simulink model "a1e1"  (R2020a)
settings: Solver=VariableStepAuto  StartTime=0.0  StopTime=200  RelTol=1e-3
settings Model: Creator=vivek vivian  LastModifiedBy=vivek vivian

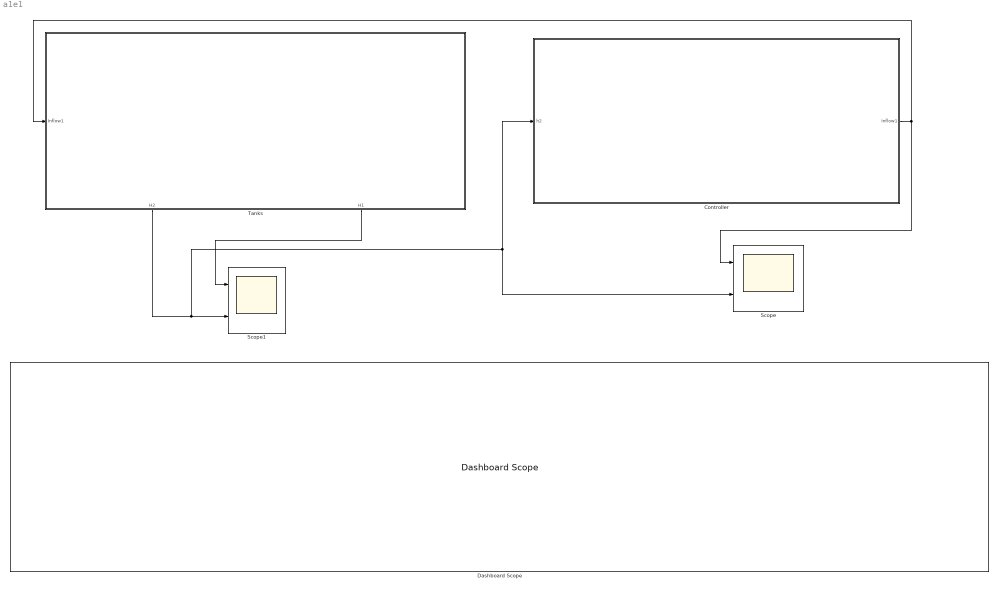
== system a1e1 ==
  Controller : Subsystem
  Dashboard Scope : DashboardScope
  Scope : Scope  NumInputPorts=2
  Scope1 : Scope  NumInputPorts=2
  Tanks : Subsystem
      settings: PortSchema="{\"entries\":[{\"content\":{\"sides\":[{\"content\":{\"connectorIds\":[\"In1\"]},\"type\":\"ConnectorPlacement.EquallySpacedRectSide\",\"uuid\":\"e5306d54-3110-4a08-a7f7-5a5ae3387896\"},{\"content\":{\"connectorIds\":[],\"side\":\"RIGHT\"},\"type\":\"ConnectorPlacement.EquallySpacedRectSide\",\"uuid\":\"42eaa8c0-5f21-4179-a706-71b62f07686c\"},{\"content\":{\"connectorIds\":[],\"side\":\"TOP\"},\"type\":\"ConnectorPlacement.EquallySpacedRectSide\",\"uuid\":\"3c777650-c00c-4d8d-89ca-bf2a69e675bf\"},{\"content\":{\"connectorIds\":[\"Out1\",\"Out2\"],\"side\":\"BOTTOM\"},\"type\":\"ConnectorPlacement.EquallySpacedRectSide\",\"uuid\":\"c8daac80-6471-486d-b612-ea006b4d9ffc\"}]},\"type\":\"ConnectorPlacement.EquallySpacedConnector\",\"uuid\":\"5a7e1e9a-909c-4566-afd0-a9330854ec0a\"}],\"packageUris\":[\"http://schema.mathworks.com/mf0/Connector/19700101\"],\"version\":\"1.0\"}"
  wires:
  Controller/1(Inflow1) -> Scope/1, Tanks/1(Inflow1)
  Tanks/1(H2) -> Scope/2, Controller/1(h2), Scope1/2
  Tanks/2(H1) -> Scope1/1

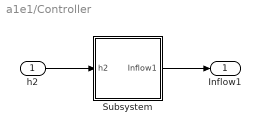
== system a1e1/Controller ==
  h2 : Inport
  Subsystem : Subsystem
  Inflow1 : Outport
  wires:
  h2/1 -> Subsystem/1(h2)
  Subsystem/1(Inflow1) -> Inflow1/1

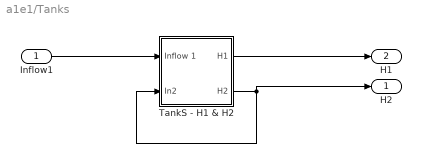
== system a1e1/Tanks ==
  Inflow1 : Inport
  TankS - H1 & H2 : Subsystem
  H2 : Outport
  H1 : Outport  Port=2
  wires:
  TankS - H1 & H2/2(H2) -> H2/1, TankS - H1 & H2/2(In2)
  Inflow1/1 -> TankS - H1 & H2/1(Inflow 1)
  TankS - H1 & H2/1(H1) -> H1/1

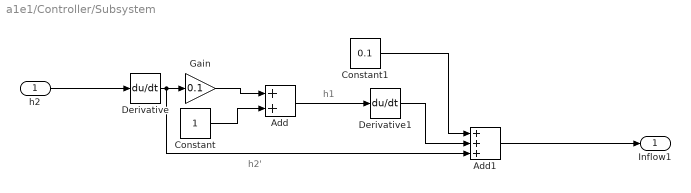
== system a1e1/Controller/Subsystem ==
  note: h2'
  note: h1
  h2 : Inport
  Add : Sum
  Add1 : Sum  Inputs=+++
  Constant : Constant
  Constant1 : Constant  Value=0.1
  Derivative : Derivative
  Derivative1 : Derivative
  Gain : Gain  Gain=0.1
  Inflow1 : Outport
  wires:
  Constant1/1 -> Add1/1
  Add1/1 -> Inflow1/1
  Derivative/1 -> Add1/3, Gain/1
  h2/1 -> Derivative/1
  Constant/1 -> Add/2
  Derivative1/1 -> Add1/2
  Gain/1 -> Add/1
  Add/1 -> Derivative1/1

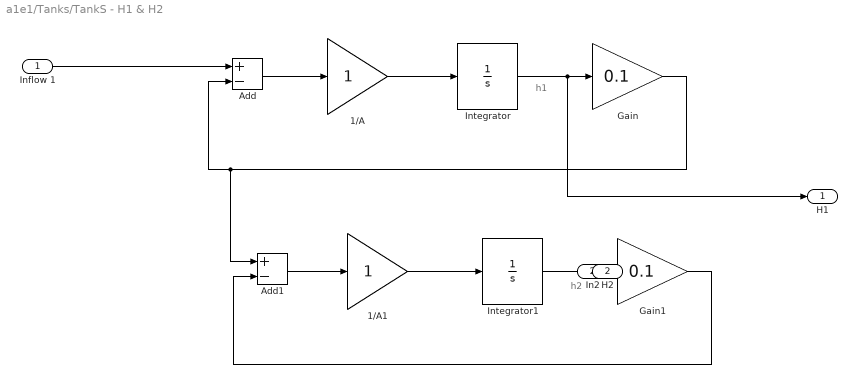
== system a1e1/Tanks/TankS - H1 & H2 ==
  note: h1
  note: h2
  Inflow 1 : Inport
  In2 : Inport  Port=2
  1/A : Gain
  1/A1 : Gain
  Add : Sum  Inputs=+-
  Add1 : Sum  Inputs=+-
  Gain : Gain  Gain=0.1
  Gain1 : Gain  Gain=0.1
  Integrator : Integrator  LowerSaturationLimit=0
  Integrator1 : Integrator  LowerSaturationLimit=0
  H1 : Outport
  H2 : Outport  Port=2
  wires:
  1/A/1 -> Integrator/1
  Integrator/1 -> H1/1, Gain/1
  Add/1 -> 1/A/1
  Gain1/1 -> Add1/2
  In2/1 -> Gain1/1
  Gain/1 -> Add1/1, Add/2
  Integrator1/1 -> H2/1
  Add1/1 -> 1/A1/1
  1/A1/1 -> Integrator1/1
  Inflow 1/1 -> Add/1
